simulink model "autopilot_controller_tuning"  (R2024b)
settings: Solver=FixedStepAuto  StartTime=0.0  StopTime=50  FixedStep=0.01  RelTol=1e-3
InitFcn:
  | %% environmental parameter
  | 
  | g = 9.81;                       %[m/ss]
  | 
  | %% Vehicle parameter
  | 
  | mass = 1.5;                     %[kg]
  | Arm_Length = 0.225;             %[m]
  | 
  | %% Motor parameter
  | 
  | rad2rpm = 60 / (2 * pi);
  | 
  | rpm2rad = 1 / rad2rpm;
  | 
  | Friction_Coef = 0.0001;         %[N m /s]
  | 
  | Inertia = 2.8e-05;              %[kg m^2]
  | 
  | Resistance = 0.1170;            %[ohm]
  | 
  | K_Torque = 1 / (rpm2rad * 960); %[N m/A]
  | 
  | K_Emf = K_Torque;               %[V s/rad]
  | 
  | tau = (Inertia * Resistance) / (Resistance * Friction_Coef + K_Torque * K_Emf);
  | 
  | k_s = K_Torque / (Resistance * Friction_Coef + K_Torque * K_Emf);
  | 
  | Thrust_Coef = 1.1768e-05;
  | 
  | Drag_Coef = 1.8542e-07;
  | 
  | Hovering_Motor_Speed = sqrt(mass * g / (4 * Thrust_Coef));
  | 
  | k_p = 1/k_s;
  | 
  | K1_ALT = 2.1;
  | K2_ALT = 0.7142;
  | 
  | K1_POS = 1.26;
  | K2_POS = 0.4286;
libraries: simulink_extras x2
settings Model: Creator=user  LastModifiedBy=user

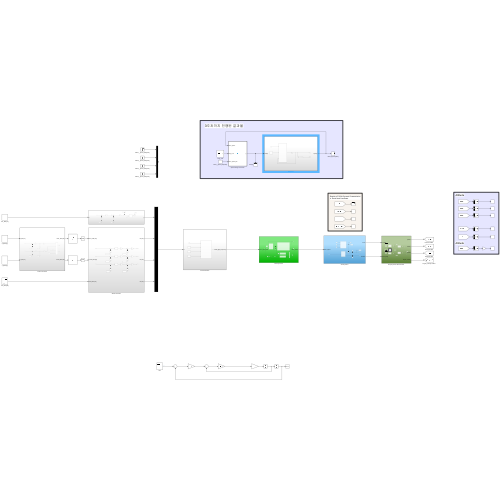
[thumbnail: Simulink's stored preview of the top-level diagram]
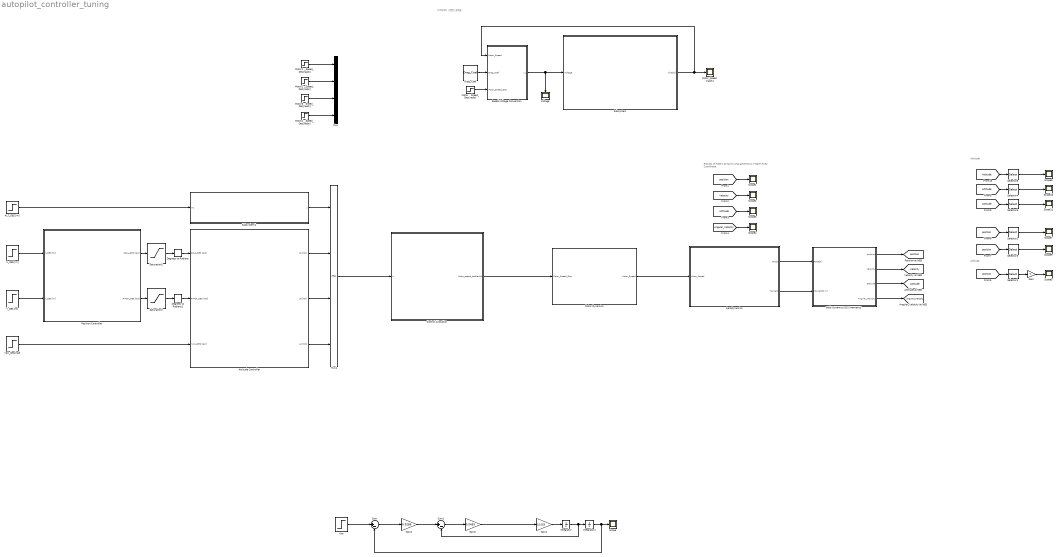
== system autopilot_controller_tuning ==
  note: Attitude
  note: Altitude
  note: Results of F450's Dynamic Characteristics
      | in Earth fixed Coordinate
  note: 3주차까지 진행된 결과물
  ALT_DES [m] : Step  After=100  SampleTime=0
  AeroDynamics : Subsystem
  Attitude Controller : Subsystem
  Body Dynamics && Kinematics : Subsystem
  Control Allocation : Subsystem
  Degrees to Radians : simulink_extras/Transformations/Degrees to Radians
  Degrees to Radians1 : simulink_extras/Transformations/Degrees to Radians
  Drag_Coef : Constant  Value=Drag_Coef
  Gain : Gain  Gain=-1
  Gain1 : Gain  Gain=0.9286
  Gain2 : Gain  Gain=0.0455
  Gain4 : Gain  Gain=1/0.025
  Integrator : Integrator
  Integrator1 : Integrator
  Motor Dynamics : Subsystem
  Motor1__Speed_Des[rad/s] : Step  Time=0  After=Hovering_Motor_Speed  SampleTime=0
  Motor2__Speed_Des[rad/s] : Step  Time=0  After=Hovering_Motor_Speed  SampleTime=0
  Motor3__Speed_Des[rad/s] : Step  Time=0  After=Hovering_Motor_Speed  SampleTime=0
  Motor4__Speed_Des[rad/s] : Step  Time=0  After=Hovering_Motor_Speed  SampleTime=0
  Motor_Speed [rad/s] : Scope
  Motor__Speed_Des[rad/s] : Step  After=Hovering_Motor_Speed  SampleTime=0
  Mux : Mux
  Mux1 : Mux
  Position Controller : Subsystem
  Saturation1 : Saturate  UpperLimit=30  LowerLimit=-30
  Saturation2 : Saturate  UpperLimit=30  LowerLimit=-30
  Scope{,1..5,7..11} (11 alike) : Scope
  Selector1 : Selector  InputPortWidth=3  IndexOptions=Index vector (dialog)  Indices=[3]  OutputSizes=1
  Selector2 : Selector  InputPortWidth=3  IndexOptions=Index vector (dialog)  Indices=1  OutputSizes=1
  Selector3 : Selector  InputPortWidth=3  IndexOptions=Index vector (dialog)  Indices=2  OutputSizes=1
  Selector4 : Selector  InputPortWidth=3  IndexOptions=Index vector (dialog)  Indices=2  OutputSizes=1
  Selector5 : Selector  InputPortWidth=3  IndexOptions=Index vector (dialog)  Indices=[3]  OutputSizes=1
  Selector8 : Selector  InputPortWidth=3  IndexOptions=Index vector (dialog)  Indices=1  OutputSizes=1
  Speed-Voltage Conversion : MATLAB Function  TreatAsAtomicUnit=on
  Subsystem : Subsystem
  Subsystem1 : Subsystem
  Sum : Sum  Inputs=|+-
  Sum1 : Sum  Inputs=|+-
  Voltage : Scope
  X_DES [m] : Step  After=-30  SampleTime=0
  Y_DES [m] : Step  After=100  SampleTime=0
  Yaw : Step  Before=160  After=-160  SampleTime=0
  Yaw_Des[rad] : Step  After=0  SampleTime=0
  tag scope: Angular_Velocity=global, Attitude=global, Velocity=global, position=global
  wires:
  Motor1__Speed_Des[rad/s]/1 -> Mux/1
  Motor2__Speed_Des[rad/s]/1 -> Mux/2
  Motor3__Speed_Des[rad/s]/1 -> Mux/3
  Motor4__Speed_Des[rad/s]/1 -> Mux/4
  Motor Dynamics/1(Motor_Speed) -> AeroDynamics/1(Motor_Speed)
  Motor__Speed_Des[rad/s]/1 -> Speed-Voltage Conversion/3(Motor_Speed_Des)
  Speed-Voltage Conversion/1(v_i) -> Voltage/1, Subsystem/1(Voltage)
  Drag_Coef/1 -> Speed-Voltage Conversion/2(Drag_Coef)
  Subsystem/1(w[rad/s]) -> Speed-Voltage Conversion/1(Motor_Speed), Motor_Speed [rad/s]/1
  Body Dynamics && Kinematics/3(attitude) -> [Attitude]
  Body Dynamics && Kinematics/1(position) -> [position]
  [Velocity] -> Scope2/1
  [position] -> Scope1/1
  AeroDynamics/1(Force) -> Body Dynamics && Kinematics/1(Force[N])
  AeroDynamics/2(Moment) -> Body Dynamics && Kinematics/2(Moment[N m])
  Body Dynamics && Kinematics/2(Velocity) -> [Velocity]
  Body Dynamics && Kinematics/4(Angular_Velocity) -> [Angular_Velocity]
  [Attitude] -> Scope3/1
  [Angular_Velocity] -> Scope4/1
  Control Allocation/1(Motor_speed_des[rad/s]) -> Motor Dynamics/1(Motor_Speed_Des)
  Mux1/1 -> Control Allocation/1(U)
  Yaw/1 -> Sum/1
  Sum/1 -> Gain1/1
  Gain1/1 -> Sum1/1
  Sum1/1 -> Gain2/1
  Gain4/1 -> Integrator/1
  Integrator/1 -> Sum1/2, Integrator1/1
  Integrator1/1 -> Sum/2, Scope/1
  Gain2/1 -> Gain4/1
  [Attitude] -> Selector8/1
  Selector8/1 -> Scope8/1
  Yaw_Des[rad]/1 -> Attitude Controller/3(YAW_DES [rad])
  Attitude Controller/1(U2 [Nm]) -> Mux1/2
  Attitude Controller/2(U3 [Nm]) -> Mux1/3
  Attitude Controller/3(U4 [Nm]) -> Mux1/4
  ALT_DES [m]/1 -> Subsystem1/1(In1)
  Subsystem1/1(y) -> Mux1/1
  Selector1/1 -> Gain/1
  Gain/1 -> Scope5/1
  X_DES [m]/1 -> Position Controller/1(X_DES [m])
  Y_DES [m]/1 -> Position Controller/2(Y_DES [m])
  [position] -> Selector1/1
  Position Controller/1(ROLL_DES [rad]) -> Saturation2/1
  Position Controller/2(PITCH_DES [rad]) -> Saturation1/1
  [position] -> Selector2/1
  Selector2/1 -> Scope7/1
  [position] -> Selector3/1
  Selector3/1 -> Scope9/1
  [Attitude] -> Selector4/1
  Selector4/1 -> Scope10/1
  [Attitude] -> Selector5/1
  Selector5/1 -> Scope11/1
  Saturation1/1 -> Degrees to Radians1/1
  Degrees to Radians1/1 -> Attitude Controller/2(PITCH_DES [rad])
  Saturation2/1 -> Degrees to Radians/1
  Degrees to Radians/1 -> Attitude Controller/1(ROLL_DES [rad])

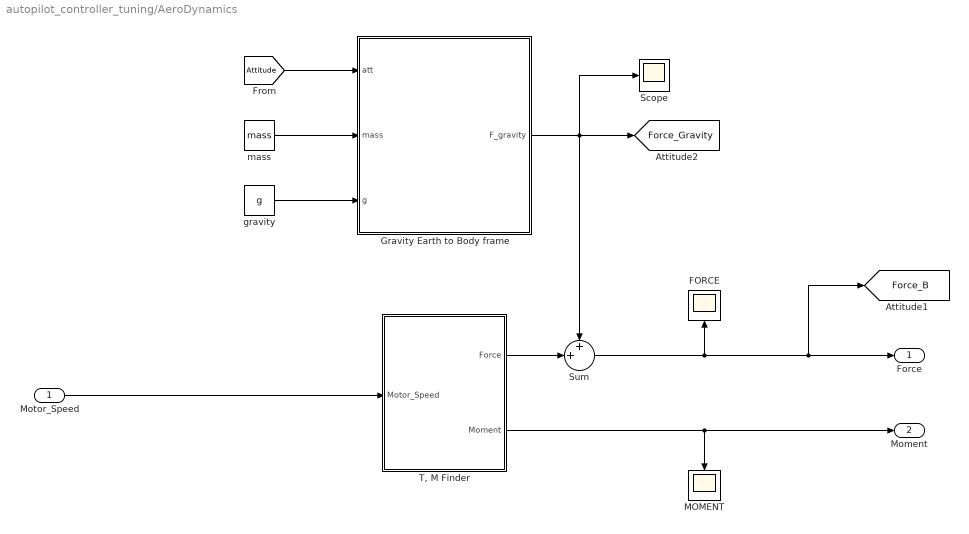
== system autopilot_controller_tuning/AeroDynamics ==
  Motor_Speed : Inport
  FORCE : Scope
  Gravity Earth to Body frame : MATLAB Function  TreatAsAtomicUnit=on
  MOMENT : Scope
  Scope : Scope
  Sum : Sum  Inputs=++|
  "T, M Finder" : MATLAB Function  TreatAsAtomicUnit=on
  gravity : Constant  Value=g
  mass : Constant  Value=mass
  Force : Outport
  Moment : Outport  Port=2
  tag scope: Force_B=global, Force_Gravity=global
  wires:
  [Attitude] -> Gravity Earth to Body frame/1(att)
  Gravity Earth to Body frame/1(F_gravity) -> Scope/1, [Force_Gravity], Sum/1
  Motor_Speed/1 -> "T, M Finder"/1(Motor_Speed)
  mass/1 -> Gravity Earth to Body frame/2(mass)
  "T, M Finder"/1(Force) -> Sum/2
  gravity/1 -> Gravity Earth to Body frame/3(g)
  Sum/1 -> [Force_B], Force/1, FORCE/1
  "T, M Finder"/2(Moment) -> Moment/1, MOMENT/1

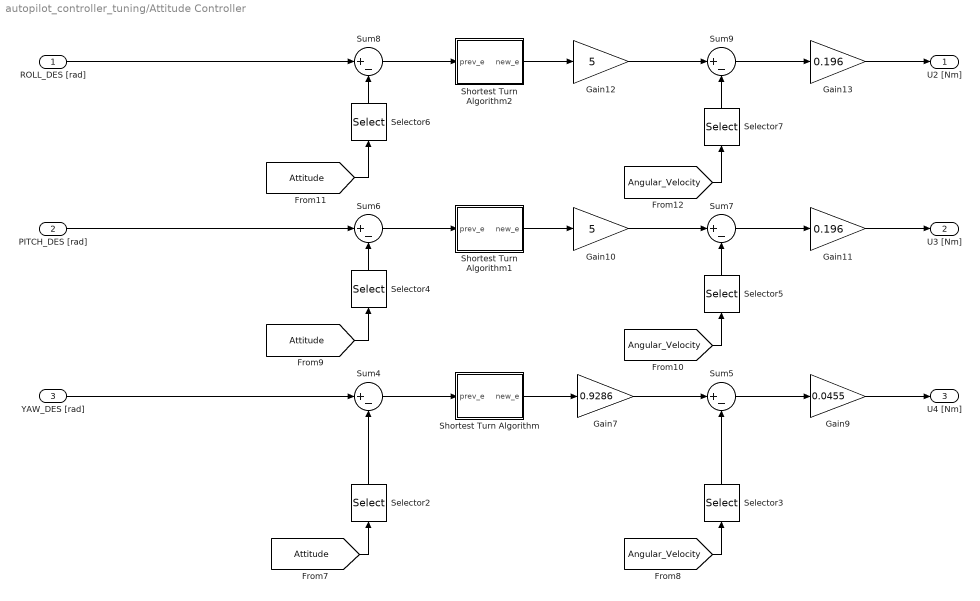
== system autopilot_controller_tuning/Attitude Controller ==
  ROLL_DES [rad] : Inport
  PITCH_DES [rad] : Inport  Port=2
  YAW_DES [rad] : Inport  Port=3
  Gain10 : Gain  Gain=5
  Gain11 : Gain  Gain=0.196
  Gain12 : Gain  Gain=5
  Gain13 : Gain  Gain=0.196
  Gain7 : Gain  Gain=0.9286
  Gain9 : Gain  Gain=0.0455
  Selector2 : Selector  InputPortWidth=3  IndexOptions=Index vector (dialog)  Indices=[3]  OutputSizes=1
  Selector3 : Selector  InputPortWidth=3  IndexOptions=Index vector (dialog)  Indices=[3]  OutputSizes=1
  Selector4 : Selector  InputPortWidth=3  IndexOptions=Index vector (dialog)  Indices=[2]  OutputSizes=1
  Selector5 : Selector  InputPortWidth=3  IndexOptions=Index vector (dialog)  Indices=[2]  OutputSizes=1
  Selector6 : Selector  InputPortWidth=3  IndexOptions=Index vector (dialog)  Indices=[1]  OutputSizes=1
  Selector7 : Selector  InputPortWidth=3  IndexOptions=Index vector (dialog)  Indices=[1]  OutputSizes=1
  Shortest Turn Algorithm : MATLAB Function  TreatAsAtomicUnit=on
  Shortest Turn Algorithm1 : MATLAB Function  TreatAsAtomicUnit=on
  Shortest Turn Algorithm2 : MATLAB Function  TreatAsAtomicUnit=on
  Sum{4..9} (6 alike) : Sum  Inputs=|+-
  U2 [Nm] : Outport
  U3 [Nm] : Outport  Port=2
  U4 [Nm] : Outport  Port=3
  wires:
  Shortest Turn Algorithm/1(new_e) -> Gain7/1
  Gain9/1 -> U4 [Nm]/1
  [Attitude] -> Selector4/1
  Selector4/1 -> Sum6/2
  [Angular_Velocity] -> Selector3/1
  Gain7/1 -> Sum5/1
  Selector6/1 -> Sum8/2
  Sum9/1 -> Gain13/1
  Gain12/1 -> Sum9/1
  Gain10/1 -> Sum7/1
  Selector5/1 -> Sum7/2
  Sum4/1 -> Shortest Turn Algorithm/1(prev_e)
  [Angular_Velocity] -> Selector7/1
  Sum7/1 -> Gain11/1
  PITCH_DES [rad]/1 -> Sum6/1
  Selector2/1 -> Sum4/2
  [Angular_Velocity] -> Selector5/1
  Gain11/1 -> U3 [Nm]/1
  Selector3/1 -> Sum5/2
  [Attitude] -> Selector6/1
  ROLL_DES [rad]/1 -> Sum8/1
  [Attitude] -> Selector2/1
  Sum5/1 -> Gain9/1
  Selector7/1 -> Sum9/2
  YAW_DES [rad]/1 -> Sum4/1
  Gain13/1 -> U2 [Nm]/1
  Sum8/1 -> Shortest Turn Algorithm2/1(prev_e)
  Shortest Turn Algorithm2/1(new_e) -> Gain12/1
  Sum6/1 -> Shortest Turn Algorithm1/1(prev_e)
  Shortest Turn Algorithm1/1(new_e) -> Gain10/1

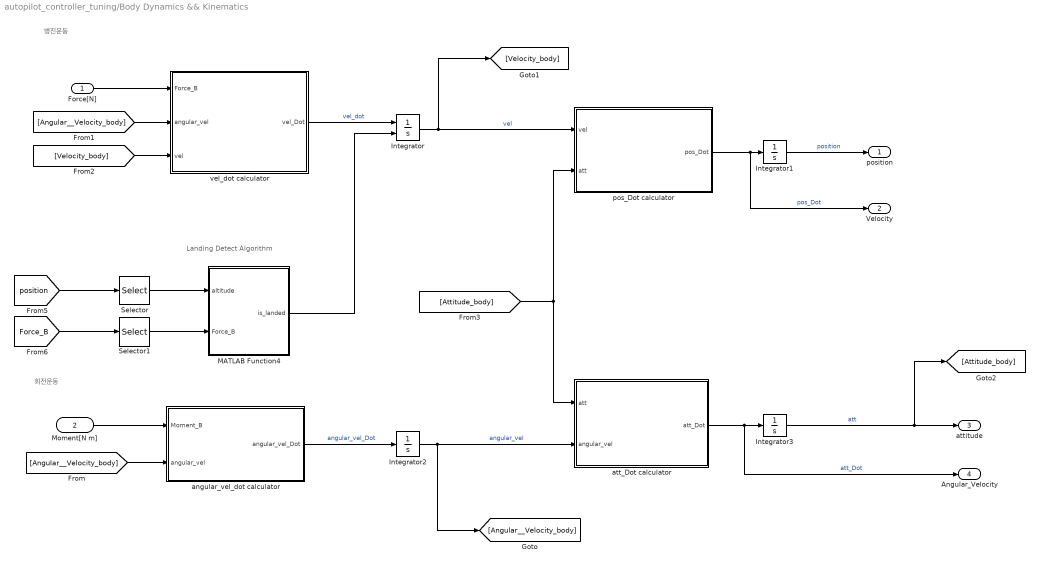
== system autopilot_controller_tuning/Body Dynamics && Kinematics ==
  note: 병진운동
  note: 회전운동
  note: Landing Detect Algorithm
  Force[N] : Inport
  Moment[N m] : Inport  Port=2
  Integrator : Integrator  ExternalReset=level hold  InitialCondition=[0 0 0]'
  Integrator1 : Integrator  InitialCondition=[0 0 0]'  LimitOutput=on  UpperSaturationLimit=[inf inf 0]'  LowerSaturationLimit=[-inf -inf -inf]'  ZeroCross=off
  Integrator2 : Integrator  InitialCondition=[0 0 0]'
  Integrator3 : Integrator  InitialCondition=[0 0 0]'  WrapState=on
  MATLAB Function4 : MATLAB Function  TreatAsAtomicUnit=on
  Selector : Selector  InputPortWidth=3  IndexOptions=Index vector (dialog)  Indices=[3]  OutputSizes=1
  Selector1 : Selector  InputPortWidth=3  IndexOptions=Index vector (dialog)  Indices=[3]  OutputSizes=1
  angular_vel_dot calculator : MATLAB Function  TreatAsAtomicUnit=on
  att_Dot calculator : MATLAB Function  TreatAsAtomicUnit=on
  pos_Dot calculator : MATLAB Function  TreatAsAtomicUnit=on
  vel_dot calculator : MATLAB Function  TreatAsAtomicUnit=on
  position : Outport
  Velocity : Outport  Port=2
  attitude : Outport  Port=3
  Angular_Velocity : Outport  Port=4
  wires:
  Force[N]/1 -> vel_dot calculator/1(Force_B)
  Moment[N m]/1 -> angular_vel_dot calculator/1(Moment_B)
  Integrator/1 -> pos_Dot calculator/1(vel), [Velocity_body]  "vel"
  pos_Dot calculator/1(pos_Dot) -> Velocity/1, Integrator1/1  "pos_Dot"
  Integrator1/1 -> position/1  "position"
  Integrator2/1 -> att_Dot calculator/2(angular_vel), [Angular__Velocity_body]  "angular_vel"
  Integrator3/1 -> attitude/1, [Attitude_body]  "att"
  att_Dot calculator/1(att_Dot) -> Angular_Velocity/1, Integrator3/1  "att_Dot"
  [Angular__Velocity_body] -> angular_vel_dot calculator/2(angular_vel)
  [Angular__Velocity_body] -> vel_dot calculator/2(angular_vel)
  [Velocity_body] -> vel_dot calculator/3(vel)
  [Attitude_body] -> pos_Dot calculator/2(att), att_Dot calculator/1(att)
  angular_vel_dot calculator/1(angular_vel_Dot) -> Integrator2/1  "angular_vel_Dot"
  vel_dot calculator/1(vel_Dot) -> Integrator/1  "vel_dot"
  MATLAB Function4/1(is_landed) -> Integrator/2
  Selector1/1 -> MATLAB Function4/2(Force_B)
  [position] -> Selector/1
  [Force_B] -> Selector1/1
  Selector/1 -> MATLAB Function4/1(altitude)

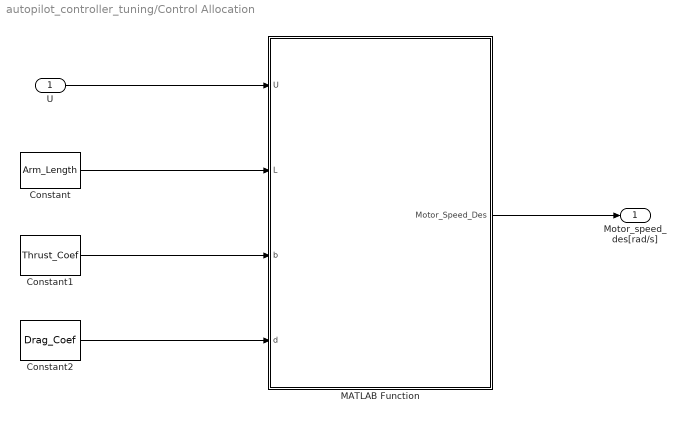
== system autopilot_controller_tuning/Control Allocation ==
  U : Inport
  Constant : Constant  Value=Arm_Length
  Constant1 : Constant  Value=Thrust_Coef
  Constant2 : Constant  Value=Drag_Coef
  MATLAB Function : MATLAB Function  TreatAsAtomicUnit=on
  Motor_speed_des[rad/s] : Outport
  wires:
  Constant2/1 -> MATLAB Function/4(d)
  MATLAB Function/1(Motor_Speed_Des) -> Motor_speed_des[rad/s]/1
  Constant1/1 -> MATLAB Function/3(b)
  Constant/1 -> MATLAB Function/2(L)
  U/1 -> MATLAB Function/1(U)

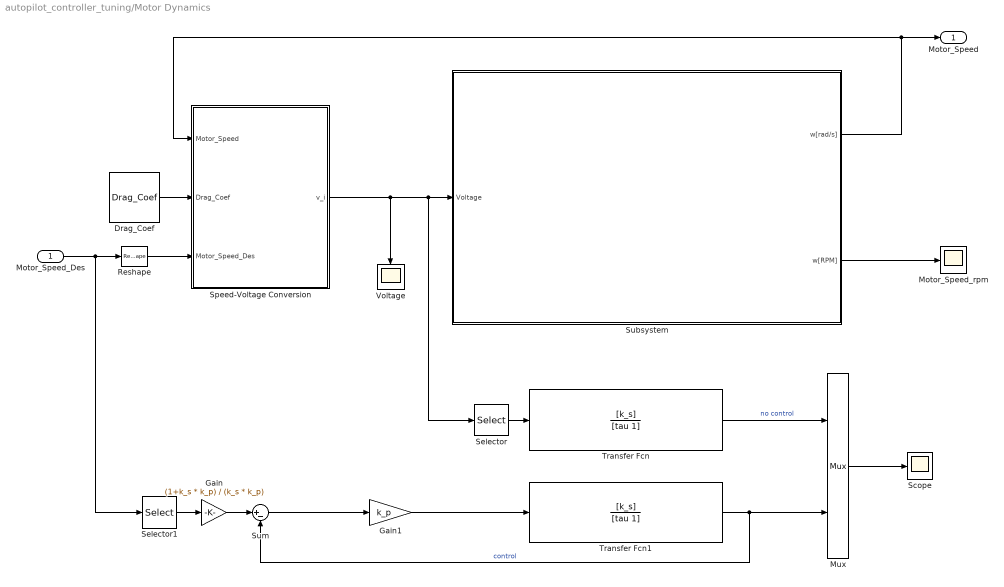
== system autopilot_controller_tuning/Motor Dynamics ==
  Motor_Speed_Des : Inport
  Drag_Coef : Constant  Value=Drag_Coef
  Gain : Gain  Gain=(1+k_s * k_p) / (k_s * k_p)
  Gain1 : Gain  Gain=k_p
  Motor_Speed_rpm : Scope
  Mux : Mux  Inputs=2
  Reshape : Reshape  OutputDimensionality=Column vector (2-D)
  Scope : Scope
  Selector : Selector  InputPortWidth=4  IndexOptions=Index vector (dialog)  Indices=1  OutputSizes=1
  Selector1 : Selector  InputPortWidth=4  IndexOptions=Index vector (dialog)  Indices=1  OutputSizes=1
  Speed-Voltage Conversion : MATLAB Function  TreatAsAtomicUnit=on
  Subsystem : Subsystem
  Sum : Sum  Inputs=|+-
  Transfer Fcn : TransferFcn  Numerator=[k_s]  Denominator=[tau 1]
  Transfer Fcn1 : TransferFcn  Numerator=[k_s]  Denominator=[tau 1]
  Voltage : Scope
  Motor_Speed : Outport
  wires:
  Speed-Voltage Conversion/1(v_i) -> Voltage/1, Subsystem/1(Voltage), Selector/1
  Drag_Coef/1 -> Speed-Voltage Conversion/2(Drag_Coef)
  Subsystem/1(w[rad/s]) -> Motor_Speed/1, Speed-Voltage Conversion/1(Motor_Speed)
  Subsystem/2(w[RPM]) -> Motor_Speed_rpm/1
  Motor_Speed_Des/1 -> Selector1/1, Reshape/1
  Reshape/1 -> Speed-Voltage Conversion/3(Motor_Speed_Des)
  Selector/1 -> Transfer Fcn/1
  Selector1/1 -> Gain/1
  Sum/1 -> Gain1/1
  Transfer Fcn1/1 -> Sum/2, Mux/2  "control"
  Gain/1 -> Sum/1
  Gain1/1 -> Transfer Fcn1/1
  Mux/1 -> Scope/1
  Transfer Fcn/1 -> Mux/1  "no control"

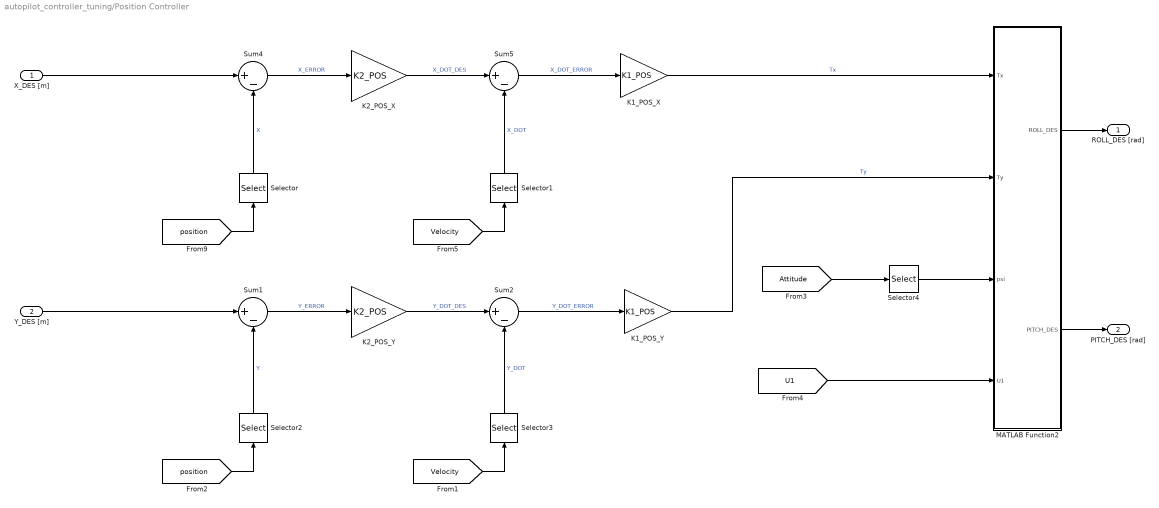
== system autopilot_controller_tuning/Position Controller ==
  X_DES [m] : Inport
  Y_DES [m] : Inport  Port=2
  K1_POS_X : Gain  Gain=K1_POS
  K1_POS_Y : Gain  Gain=K1_POS
  K2_POS_X : Gain  Gain=K2_POS
  K2_POS_Y : Gain  Gain=K2_POS
  MATLAB Function2 : MATLAB Function  TreatAsAtomicUnit=on
  Selector : Selector  InputPortWidth=3  IndexOptions=Index vector (dialog)  Indices=1  OutputSizes=1
  Selector1 : Selector  InputPortWidth=3  IndexOptions=Index vector (dialog)  Indices=1  OutputSizes=1
  Selector2 : Selector  InputPortWidth=3  IndexOptions=Index vector (dialog)  Indices=2  OutputSizes=1
  Selector3 : Selector  InputPortWidth=3  IndexOptions=Index vector (dialog)  Indices=2  OutputSizes=1
  Selector4 : Selector  InputPortWidth=3  IndexOptions=Index vector (dialog)  Indices=3  OutputSizes=1
  Sum{1..2,4..5} (4 alike) : Sum  Inputs=|+-
  ROLL_DES [rad] : Outport
  PITCH_DES [rad] : Outport  Port=2
  wires:
  [position] -> Selector/1
  K1_POS_X/1 -> MATLAB Function2/1(Tx)  "Tx"
  X_DES [m]/1 -> Sum4/1
  Selector/1 -> Sum4/2  "X"
  [Velocity] -> Selector1/1
  Sum5/1 -> K1_POS_X/1  "X_DOT_ERROR"
  Selector1/1 -> Sum5/2  "X_DOT"
  K2_POS_X/1 -> Sum5/1  "X_DOT_DES"
  Sum4/1 -> K2_POS_X/1  "X_ERROR"
  [position] -> Selector2/1
  K1_POS_Y/1 -> MATLAB Function2/2(Ty)  "Ty"
  Y_DES [m]/1 -> Sum1/1
  Selector2/1 -> Sum1/2  "Y"
  [Velocity] -> Selector3/1
  Sum2/1 -> K1_POS_Y/1  "Y_DOT_ERROR"
  Selector3/1 -> Sum2/2  "Y_DOT"
  K2_POS_Y/1 -> Sum2/1  "Y_DOT_DES"
  Sum1/1 -> K2_POS_Y/1  "Y_ERROR"
  [Attitude] -> Selector4/1
  Selector4/1 -> MATLAB Function2/3(psi)
  [U1] -> MATLAB Function2/4(U1)
  MATLAB Function2/1(ROLL_DES) -> ROLL_DES [rad]/1
  MATLAB Function2/2(PITCH_DES) -> PITCH_DES [rad]/1

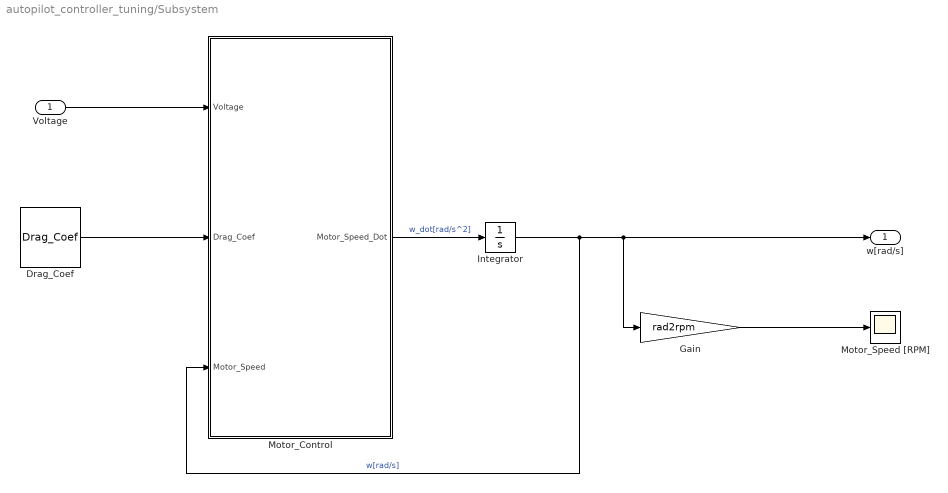
== system autopilot_controller_tuning/Subsystem ==
  Voltage : Inport
  Drag_Coef : Constant  Value=Drag_Coef
  Gain : Gain  Gain=rad2rpm
  Integrator : Integrator
  Motor_Control : MATLAB Function  TreatAsAtomicUnit=on
  Motor_Speed [RPM] : Scope
  w[rad/s] : Outport
  wires:
  Motor_Control/1(Motor_Speed_Dot) -> Integrator/1  "w_dot[rad/s^2]"
  Integrator/1 -> w[rad/s]/1, Gain/1, Motor_Control/3(Motor_Speed)  "w[rad/s]"
  Gain/1 -> Motor_Speed [RPM]/1
  Voltage/1 -> Motor_Control/1(Voltage)
  Drag_Coef/1 -> Motor_Control/2(Drag_Coef)

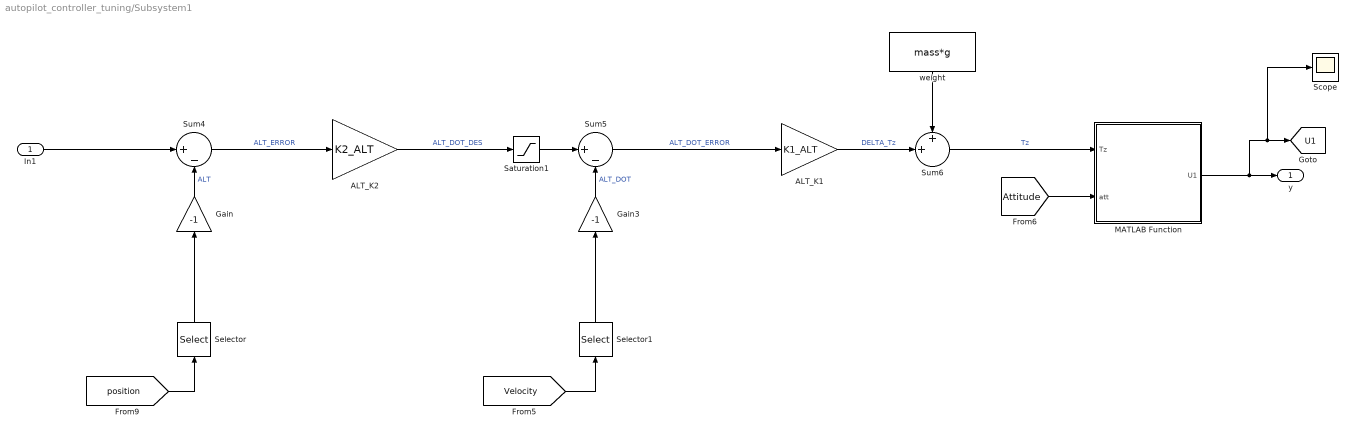
== system autopilot_controller_tuning/Subsystem1 ==
  In1 : Inport
  ALT_K1 : Gain  Gain=K1_ALT
  ALT_K2 : Gain  Gain=K2_ALT
  Gain : Gain  Gain=-1
  Gain3 : Gain  Gain=-1
  MATLAB Function : MATLAB Function  TreatAsAtomicUnit=on
  Saturation1 : Saturate  UpperLimit=3  LowerLimit=-1.5
  Scope : Scope
  Selector : Selector  InputPortWidth=3  IndexOptions=Index vector (dialog)  Indices=3  OutputSizes=1
  Selector1 : Selector  InputPortWidth=3  IndexOptions=Index vector (dialog)  Indices=3  OutputSizes=1
  Sum4 : Sum  Inputs=|+-
  Sum5 : Sum  Inputs=|+-
  Sum6 : Sum  Inputs=++|
  weight : Constant  Value=mass*g
  y : Outport
  tag scope: U1=global
  wires:
  Gain3/1 -> Sum5/2  "ALT_DOT"
  Sum5/1 -> ALT_K1/1  "ALT_DOT_ERROR"
  ALT_K2/1 -> Saturation1/1  "ALT_DOT_DES"
  Sum4/1 -> ALT_K2/1  "ALT_ERROR"
  Sum6/1 -> MATLAB Function/1(Tz)  "Tz"
  weight/1 -> Sum6/1
  ALT_K1/1 -> Sum6/2  "DELTA_Tz"
  Selector1/1 -> Gain3/1
  [position] -> Selector/1
  Gain/1 -> Sum4/2  "ALT"
  Selector/1 -> Gain/1
  [Velocity] -> Selector1/1
  [Attitude] -> MATLAB Function/2(att)
  MATLAB Function/1(U1) -> Scope/1, [U1], y/1
  In1/1 -> Sum4/1
  Saturation1/1 -> Sum5/1

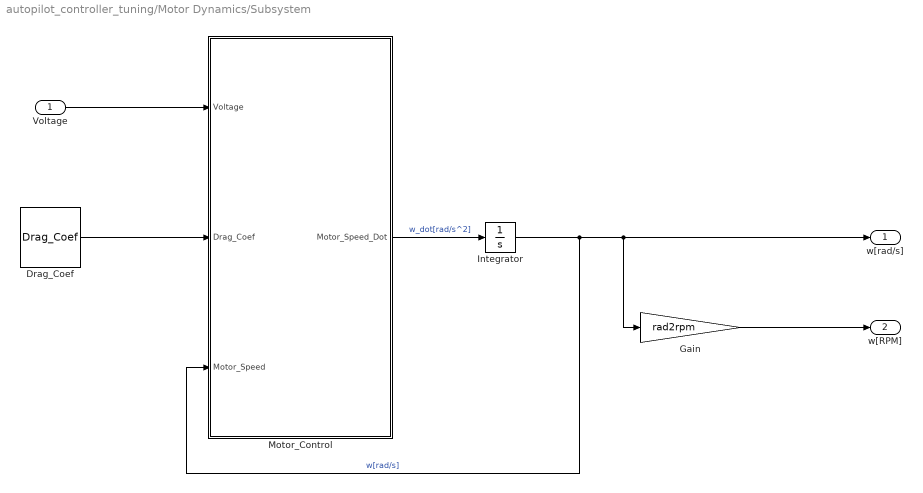
== system autopilot_controller_tuning/Motor Dynamics/Subsystem ==
  Voltage : Inport
  Drag_Coef : Constant  Value=Drag_Coef
  Gain : Gain  Gain=rad2rpm
  Integrator : Integrator  InitialCondition=[0 0 0 0]'
  Motor_Control : MATLAB Function  TreatAsAtomicUnit=on
  w[rad/s] : Outport
  w[RPM] : Outport  Port=2
  wires:
  Motor_Control/1(Motor_Speed_Dot) -> Integrator/1  "w_dot[rad/s^2]"
  Integrator/1 -> w[rad/s]/1, Gain/1, Motor_Control/3(Motor_Speed)  "w[rad/s]"
  Gain/1 -> w[RPM]/1
  Voltage/1 -> Motor_Control/1(Voltage)
  Drag_Coef/1 -> Motor_Control/2(Drag_Coef)

== matlab function autopilot_controller_tuning/Body Dynamics && Kinematics/MATLAB Function4 ==
  data: is_landed output; altitude input; Force_B input
function is_landed = fcn(altitude, Force_B)

is_landed = (altitude >= 0) && (Force_B > 0);

end

== matlab function autopilot_controller_tuning/Attitude Controller/Shortest Turn Algorithm ==
  data: prev_e input; new_e output
function new_e = fcn(prev_e)

if prev_e > pi
    new_e = prev_e - 2 * pi;
elseif prev_e < -pi
    new_e = prev_e + 2 * pi;
else
    new_e = prev_e;
end

== matlab function autopilot_controller_tuning/Attitude Controller/Shortest Turn Algorithm1 ==
  data: prev_e input; new_e output
function new_e = fcn(prev_e)

if prev_e > pi
    new_e = prev_e - 2 * pi;
elseif prev_e < -pi
    new_e = prev_e + 2 * pi;
else
    new_e = prev_e;
end

== matlab function autopilot_controller_tuning/Attitude Controller/Shortest Turn Algorithm2 ==
  data: prev_e input; new_e output
function new_e = fcn(prev_e)

if prev_e > pi
    new_e = prev_e - 2 * pi;
elseif prev_e < -pi
    new_e = prev_e + 2 * pi;
else
    new_e = prev_e;
end

== matlab function autopilot_controller_tuning/Control Allocation/MATLAB Function ==
  data: U input; Motor_Speed_Des output; L input; b input; d input
function Motor_Speed_Des = fcn(U, L, b, d)

lb = L*b/sqrt(2);


%Arm이 +일 때
%AC = [b  b  b  b;
%      0 -lb 0 lb;
%      lb 0 -lb 0;
%      -d d -d d] ^ (-1);


%Arm이 x일 때
AC = [b  b  b  b;
      -lb lb lb -lb;
      lb -lb lb -lb;
      d d -d -d] ^ (-1);

Motor_Speed_Des_2 = max(AC * U, 0);

Motor_Speed_Des = sqrt(Motor_Speed_Des_2);

== matlab function autopilot_controller_tuning/Subsystem1/MATLAB Function ==
  data: Tz input; U1 output; att input
function U1 = fcn(Tz, att)

phi = att(1);
theta = att(2);

U1 = Tz / (cos(phi) * cos(theta));

end

== matlab function autopilot_controller_tuning/Position Controller/MATLAB Function2 ==
  data: Tx input; ROLL_DES output; Ty input; psi input; U1 input; PITCH_DES output
function [ROLL_DES, PITCH_DES] = fcn(Tx, Ty, psi, U1)

Txx = Tx * cos(psi) + Ty * sin(psi);     %Tx'
Tyy = -Tx * sin(psi) + Ty * cos(psi);    %Ty'


ROLL_DES = Tyy/U1;
PITCH_DES = -Txx/U1;

== matlab function autopilot_controller_tuning/Motor Dynamics/Speed-Voltage Conversion ==
  data: Motor_Speed input; Drag_Coef input; Motor_Speed_Des input; v_i output
function v_i = fcn(Motor_Speed, Drag_Coef, Motor_Speed_Des)

rad2rpm = 60 / (2 * pi);

rpm2rad = 1 / rad2rpm;

Resistance = 0.1170;            %[ohm]

K_Torque = 1 / (rpm2rad * 960); %[N m/A]

K_Emf = K_Torque;               %[V s/rad]


v_i = K_Emf .* Motor_Speed_Des + Resistance/K_Torque * Drag_Coef .* Motor_Speed.^2;


end

== matlab function autopilot_controller_tuning/Motor Dynamics/Subsystem/Motor_Control ==
  data: Voltage input; Drag_Coef input; Motor_Speed_Dot output; Motor_Speed input
function Motor_Speed_Dot = fcn(Voltage, Drag_Coef, Motor_Speed)

rad2rpm = 60 / (2 * pi);

rpm2rad = 1 / rad2rpm;

Inertia = 2.8e-05;              %[kg m^2]

Resistance = 0.1170;            %[ohm]

K_Torque = 1 / (rpm2rad * 960); %[N m/A]

K_Emf = K_Torque;               %[V s/rad]

V_Emf = K_Emf .* Motor_Speed; %[Voltage]

Current = (Voltage - V_Emf) / Resistance; %[A]

Motor_Speed_Dot = (K_Torque * Current - Drag_Coef * Motor_Speed.^2)/ Inertia; %[rad/s^2]

end

== matlab function autopilot_controller_tuning/AeroDynamics/T, M Finder ==
  data: Motor_Speed input; Force output; Moment output
function [Force, Moment] = fcn(Motor_Speed)

Thrust_Coef = 1.1768e-05;

Drag_Coef = 1.8542e-07;

Arm_Length = 0.225;             %[m]


Force = [0;
         0;
         -Thrust_Coef * sum(Motor_Speed.^2)];


%% Cal Moment
Mx = Arm_Length * Thrust_Coef * (Motor_Speed(3)^2 + Motor_Speed(2)^2 - Motor_Speed(1)^2 -Motor_Speed(4)^2) / sqrt(2);
My = Arm_Length * Thrust_Coef * (Motor_Speed(1)^2 + Motor_Speed(3)^2 - Motor_Speed(2)^2 - Motor_Speed(4)^2) / sqrt(2);
Mz = Drag_Coef * (Motor_Speed(1)^2 + Motor_Speed(2)^2 - Motor_Speed(3)^2 - Motor_Speed(4)^2);

Moment = [Mx; My; Mz];

== matlab function autopilot_controller_tuning/Speed-Voltage Conversion ==
  data: Motor_Speed input; Drag_Coef input; Motor_Speed_Des input; v_i output
function v_i = fcn(Motor_Speed, Drag_Coef, Motor_Speed_Des)

rad2rpm = 60 / (2 * pi);

rpm2rad = 1 / rad2rpm;

Resistance = 0.1170;            %[ohm]

K_Torque = 1 / (rpm2rad * 960); %[N m/A]

K_Emf = K_Torque;               %[V s/rad]


v_i = K_Emf * Motor_Speed_Des + Resistance/K_Torque * Drag_Coef * Motor_Speed^2;


end

== matlab function autopilot_controller_tuning/Subsystem/Motor_Control ==
  data: Voltage input; Drag_Coef input; Motor_Speed_Dot output; Motor_Speed input
function Motor_Speed_Dot = fcn(Voltage, Drag_Coef, Motor_Speed)

rad2rpm = 60 / (2 * pi);

rpm2rad = 1 / rad2rpm;

Inertia = 2.8e-05;              %[kg m^2]

Resistance = 0.1170;            %[ohm]

K_Torque = 1 / (rpm2rad * 960); %[N m/A]

K_Emf = K_Torque;               %[V s/rad]

V_Emf = K_Emf * Motor_Speed; %[Voltage]

Current = (Voltage - V_Emf) / Resistance; %[A]

Motor_Speed_Dot = (K_Torque * Current - Drag_Coef * Motor_Speed^2)/ Inertia; %[rad/s^2]

end

== matlab function autopilot_controller_tuning/AeroDynamics/Gravity Earth to Body frame ==
  data: att input; F_gravity output; mass input; g input
function F_gravity = fcn(att, mass, g)

phi = att(1);
theta = att(2);

gravity = g * [-sin(theta);
                sin(phi)*cos(theta);
                cos(phi)*cos(theta)];

F_gravity = mass * gravity;

== matlab function autopilot_controller_tuning/Body Dynamics && Kinematics/vel_dot calculator ==
  data: Force_B input; vel_Dot output; angular_vel input; vel input
function vel_Dot = fcn(Force_B, angular_vel, vel)
mass = 1.5;
vel_Dot = Force_B / mass - cross(angular_vel, vel);

== matlab function autopilot_controller_tuning/Body Dynamics && Kinematics/angular_vel_dot calculator ==
  data: Moment_B input; angular_vel_Dot output; angular_vel input
function angular_vel_Dot = fcn(Moment_B, angular_vel)

Inertia = diag([0.02 0.02 0.025]);

angular_vel_Dot = Inertia ^ (-1) * (Moment_B - cross(angular_vel, Inertia * angular_vel));

== matlab function autopilot_controller_tuning/Body Dynamics && Kinematics/pos_Dot calculator ==
  data: vel input; pos_Dot output; att input
function pos_Dot = fcn(vel, att)
%바디축의 velocity

phi = att(1);
theta = att(2);
psi = att(3);

c_psi = cos(psi);
s_psi = sin(psi);
c_theta = cos(theta);
s_theta = sin(theta);
c_phi = cos(phi);
s_phi = sin(phi);


%R_EB
R_B2E = [c_psi*c_theta      c_psi*s_theta*s_phi-s_psi*c_phi         c_psi*s_theta*c_phi + s_psi*s_phi;
        s_psi*c_theta       s_psi*s_theta*s_phi + c_psi*c_phi       s_psi*s_theta*c_phi - c_psi*s_phi;
           -s_theta                 c_theta*s_phi                               c_theta*c_phi];



pos_Dot = R_B2E * vel;

== matlab function autopilot_controller_tuning/Body Dynamics && Kinematics/att_Dot calculator ==
  data: att input; angular_vel input; att_Dot output
function att_Dot = fcn(att, angular_vel)

phi = att(1);
theta = att(2);



R_B2E = [1      sin(phi)*tan(theta)     cos(phi)*tan(theta);
         0              cos(phi)            -sin(phi);
         0      sin(phi)*sec(theta)     cos(phi)*sec(theta)];


att_Dot = R_B2E * angular_vel;
